simulink model "daolibai_2016b"  (R2016b)
settings: Solver=VariableStepAuto  StartTime=0.0  StopTime=60  RelTol=1e-3
values from neighbouring files (symbols this model uses):
  AKD = 0.05    [RUN2016b.m]
  AKI = 0.12    [RUN2016b.m]
  AKP = 0.25    [RUN2016b.m]
  b = 0.1    [RUN2016b.m]
  dF = 1    [RUN2016b.m]
  g = 9.81    [RUN2016b.m]
  I = 0.006    [RUN2016b.m]
  l = 0.3    [RUN2016b.m]
  m = 0.2    [RUN2016b.m]
  M = 0.5    [RUN2016b.m]
  PKD = 1    [RUN2016b.m]
  PKI = 0.0    (= 0)    [RUN2016b.m]
  PKP = 1    [RUN2016b.m]
  theta_0 = 150*pi/180    (= 2.61799387799)    [RUN2016b.m]
libraries: aerolibconvert2 x1
settings Model: Creator=90713  LastModifiedBy=90713
settings DebuggingCC: UnconnectedInputMsg=none  UnconnectedOutputMsg=none  UnconnectedLineMsg=none  SFMachineParentedDataDiag=error
settings SFSimCC: SimUseLocalCustomCode=on
settings RTWCC: RTWUseLocalCustomCode=on

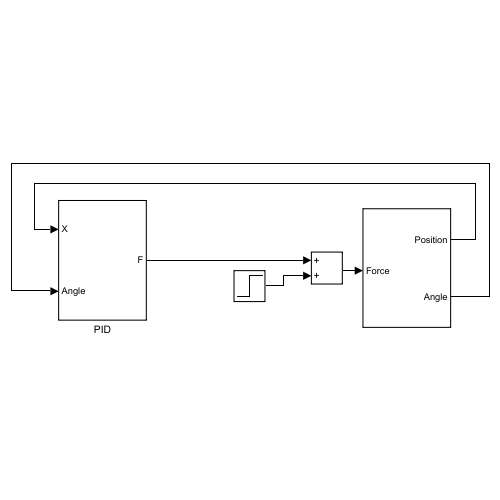
[thumbnail: Simulink's stored preview of the top-level diagram]
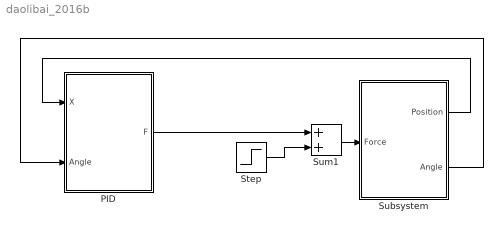
== system daolibai_2016b ==
  PID : Subsystem
  Step : Step  Time=20  After=dF  SampleTime=1
  Subsystem : Subsystem
  Sum1 : Sum
  wires:
  Step/1 -> Sum1/2
  Subsystem/2(Angle) -> PID/2(Angle)
  Subsystem/1(Position) -> PID/1(X)
  PID/1(F) -> Sum1/1
  Sum1/1 -> Subsystem/1(Force)

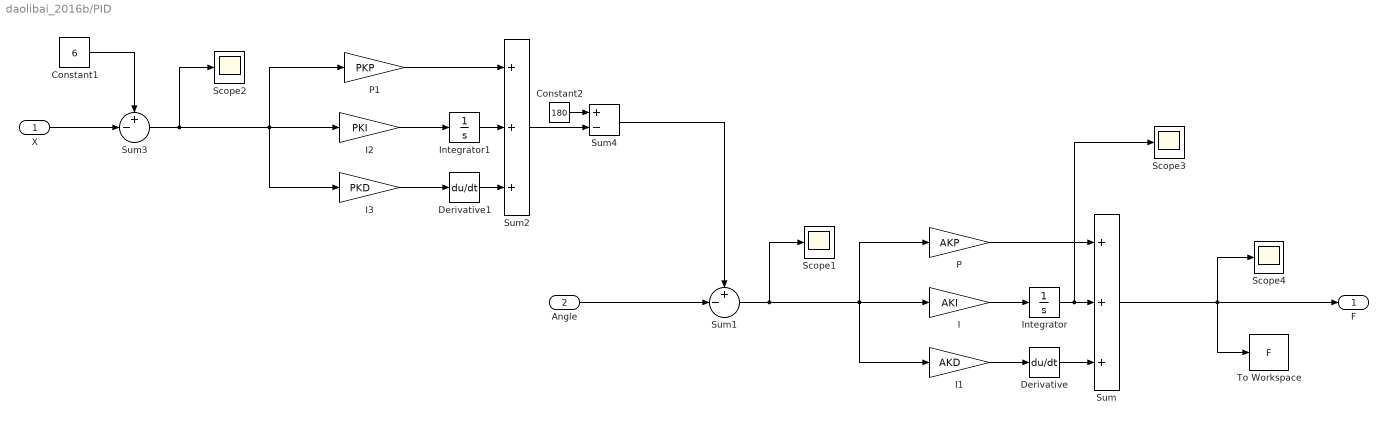
== system daolibai_2016b/PID ==
  X : Inport
  Angle : Inport  Port=2
  Constant1 : Constant  Value=6
  Constant2 : Constant  Value=180
  Derivative : Derivative
  Derivative1 : Derivative
  I : Gain  Gain=AKI
  I1 : Gain  Gain=AKD
  I2 : Gain  Gain=PKI
  I3 : Gain  Gain=PKD
  Integrator : Integrator  LimitOutput=on  UpperSaturationLimit=400  LowerSaturationLimit=-400
  Integrator1 : Integrator  LimitOutput=on  UpperSaturationLimit=400  LowerSaturationLimit=-400
  P : Gain  Gain=AKP
  P1 : Gain  Gain=PKP
  Scope{1..4} (4 alike) : Scope
  Sum : Sum  Inputs=+++
  Sum1 : Sum  Inputs=+-|
  Sum2 : Sum  Inputs=+++
  Sum3 : Sum  Inputs=+-|
  Sum4 : Sum  Inputs=+-
  To Workspace : ToWorkspace  VariableName=F  SampleTime=-1
  F : Outport
  wires:
  I/1 -> Integrator/1
  I1/1 -> Derivative/1
  Derivative/1 -> Sum/3
  P/1 -> Sum/1
  Integrator/1 -> Scope3/1, Sum/2
  Sum/1 -> To Workspace/1, F/1, Scope4/1
  Sum1/1 -> Scope1/1, I1/1, P/1, I/1
  P1/1 -> Sum2/1
  Integrator1/1 -> Sum2/2
  Derivative1/1 -> Sum2/3
  I2/1 -> Integrator1/1
  Sum3/1 -> Scope2/1, I3/1, P1/1, I2/1
  X/1 -> Sum3/2
  I3/1 -> Derivative1/1
  Sum2/1 -> Sum4/2
  Constant2/1 -> Sum4/1
  Constant1/1 -> Sum3/1
  Sum4/1 -> Sum1/1
  Angle/1 -> Sum1/2

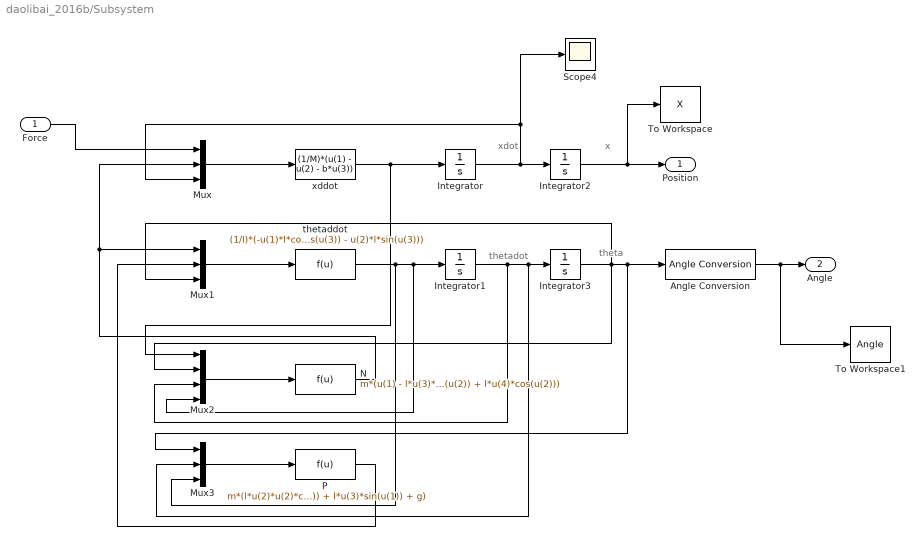
== system daolibai_2016b/Subsystem ==
  note: theta
  note: x
  note: thetadot
  note: xdot
  Force : Inport
  Angle Conversion : aerolibconvert2/Angle Conversion  IU=rad  OU=deg
  Integrator : Integrator  ContinuousStateAttributes='xdot'
  Integrator1 : Integrator  ContinuousStateAttributes='thetadot'
  Integrator2 : Integrator  ContinuousStateAttributes='x'
  Integrator3 : Integrator  InitialCondition=theta_0  ContinuousStateAttributes='theta'
  Mux : Mux  Inputs=3
  Mux1 : Mux  Inputs=3
  Mux2 : Mux
  Mux3 : Mux  Inputs=3
  N : Fcn  Expr=m*(u(1) - l*u(3)*u(3)*sin(u(2)) + l*u(4)*cos(u(2)))
  P : Fcn  Expr=m*(l*u(2)*u(2)*cos(u(1)) + l*u(3)*sin(u(1)) + g)
  Scope4 : Scope
  To Workspace : ToWorkspace  VariableName=X  SaveFormat=Timeseries  SampleTime=-1
  To Workspace1 : ToWorkspace  VariableName=Angle  SaveFormat=Timeseries  SampleTime=-1
  thetaddot : Fcn  Expr=(1/I)*(-u(1)*l*cos(u(3)) - u(2)*l*sin(u(3)))
  xddot : Fcn  Expr=(1/M)*(u(1) - u(2) - b*u(3))
  Position : Outport
  Angle : Outport  Port=2
  wires:
  Force/1 -> Mux/1
  Mux2/1 -> N/1
  Mux/1 -> xddot/1
  P/1 -> Mux1/2
  Mux3/1 -> P/1
  N/1 -> Mux1/1, Mux/2
  Mux1/1 -> thetaddot/1
  xddot/1 -> Mux2/1, Integrator/1
  Integrator2/1 -> To Workspace/1, Position/1
  thetaddot/1 -> Mux3/3, Mux2/4, Integrator1/1
  Integrator/1 -> Scope4/1, Mux/3, Integrator2/1
  Integrator1/1 -> Mux2/3, Mux3/2, Integrator3/1
  Integrator3/1 -> Mux2/2, Mux1/3, Angle Conversion/1, Mux3/1
  Angle Conversion/1 -> To Workspace1/1, Angle/1
